simulink model "SimulinkConcepts"  (R2018b)
settings: Solver=FixedStepDiscrete  StartTime=0.0  StopTime=20  FixedStep=1  RelTol=1e-3
model workspace (MAT data in the model file):
  a = 1
settings Model: Creator=vk09330  LastModifiedBy=vk09330
settings SFSimCC: SimUseLocalCustomCode=off
settings RTWCC: RTWUseLocalCustomCode=off

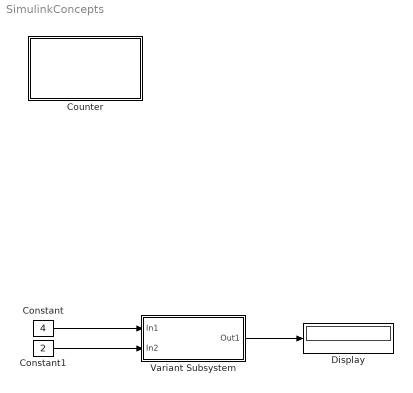
== system SimulinkConcepts ==
  Constant : Constant  Value=4
  Constant1 : Constant  Value=2
  Counter : Subsystem
  Display : Display
  Variant Subsystem : Subsystem  Variant=on
  wires:
  Variant Subsystem/1(Out1) -> Display/1
  Constant/1 -> Variant Subsystem/1(In1)
  Constant1/1 -> Variant Subsystem/2(In2)

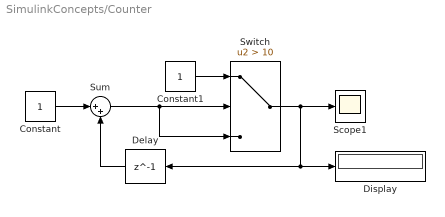
== system SimulinkConcepts/Counter ==
  Constant : Constant
  Constant1 : Constant
  Delay : Delay  DelayLength=1
  Display : Display
  Scope1 : Scope
  Sum : Sum  Inputs=|++
  Switch : Switch  Criteria=u2 > Threshold  Threshold=10
  wires:
  Constant1/1 -> Switch/1
  Constant/1 -> Sum/1
  Delay/1 -> Sum/2
  Sum/1 -> Switch/3, Switch/2
  Switch/1 -> Display/1, Delay/1, Scope1/1

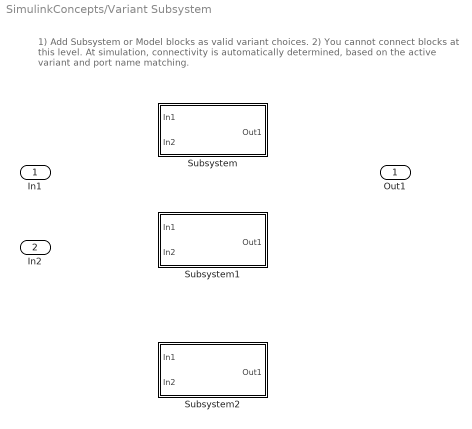
== system SimulinkConcepts/Variant Subsystem ==
  note: 1) Add Subsystem or Model blocks as valid variant choices.
      | 2) You cannot connect blocks at this level. At simulation, connectivity is automatically
      | determined, based on the active variant and port name matching.
  In1 : Inport
  In2 : Inport  Port=2
  Subsystem : Subsystem  VariantControl=a==1
  Subsystem1 : Subsystem  VariantControl=a==2
  Subsystem2 : Subsystem  VariantControl=a==3
  Out1 : Outport

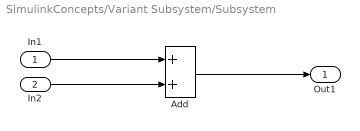
== system SimulinkConcepts/Variant Subsystem/Subsystem ==
  In1 : Inport
  In2 : Inport  Port=2
  Add : Sum
  Out1 : Outport
  wires:
  In1/1 -> Add/1
  Add/1 -> Out1/1
  In2/1 -> Add/2

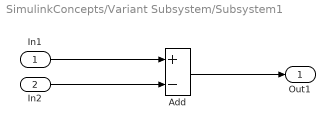
== system SimulinkConcepts/Variant Subsystem/Subsystem1 ==
  In1 : Inport
  In2 : Inport  Port=2
  Add : Sum  Inputs=+-
  Out1 : Outport
  wires:
  Add/1 -> Out1/1
  In2/1 -> Add/2
  In1/1 -> Add/1

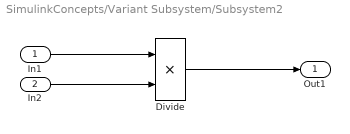
== system SimulinkConcepts/Variant Subsystem/Subsystem2 ==
  In1 : Inport
  In2 : Inport  Port=2
  Divide : Product  Inputs=**
  Out1 : Outport
  wires:
  In1/1 -> Divide/1
  Divide/1 -> Out1/1
  In2/1 -> Divide/2
